simulink model "my_model"  (R2019a)
settings: Solver=VariableStepAuto  StartTime=0.0  StopTime=10.0  RelTol=1e-3
values from neighbouring files (symbols this model uses):
  i = ii(p)    [mom.m]
  j = jj(q)    [mom.m]
settings Model: Creator=SHASHANK RAJPUT  LastModifiedBy=SHASHANK RAJPUT

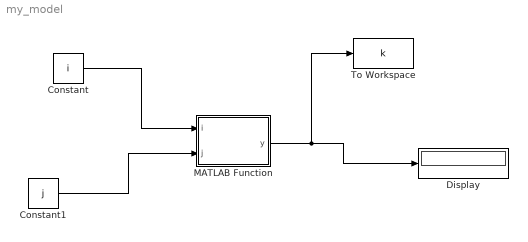
== system my_model ==
  Constant : Constant  Value=i
  Constant1 : Constant  Value=j
  Display : Display
  MATLAB Function : MATLAB Function  TreatAsAtomicUnit=on
  To Workspace : ToWorkspace  VariableName=k  SaveFormat=Timeseries  SampleTime=-1
  wires:
  Constant/1 -> MATLAB Function/1(i)
  Constant1/1 -> MATLAB Function/2(j)
  MATLAB Function/1(y) -> To Workspace/1, Display/1

== matlab function my_model/MATLAB Function ==
  data: i input; y output; j input
function y = my_model(i,j)


y = i+j;
